simulink model "TransmissionController"  (Simulink 7.6)
settings: Solver=ode45  StartTime=0.0  StopTime=10.0  RelTol=1e-3
libraries: simulink x1
settings Model: Creator=Zsolt  LastModifiedBy=bapty
settings HardwareCC: TargetIntDivRoundTo=Zero  TargetEndianess=LittleEndian  TargetHWDeviceType=MATLAB Host  ProdEqTarget=off
settings RTWCC: SystemTargetFile=rsim.tlc  TemplateMakefile=rsim_default_tmf  Description=Rapid Simulation Target  ProcessScript=rsim_make_rtw_hook
settings RSimTargetCC: TargetFunctionLibrary=ANSI_C  ERTMultiwordTypeDef=System defined  ERTCodeCoverageTool=None  ERTMultiwordLength=256  IsPILTarget=off  EnableShiftOperators=on  PortableWordSizes=off

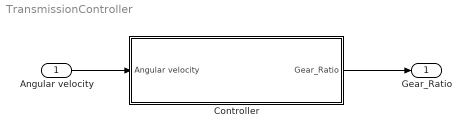
== system TransmissionController ==
  Angular velocity : Inport
  Controller : Subsystem
  Gear_Ratio : Outport
  wires:
  Angular velocity/1 -> Controller/1(Angular velocity)
  Controller/1(Gear_Ratio) -> Gear_Ratio/1

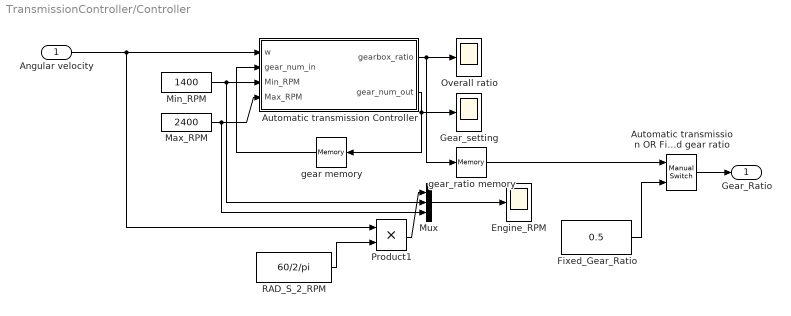
== system TransmissionController/Controller ==
  Angular velocity : Inport
  Automatic transmission Controller : Stateflow chart  TreatAsAtomicUnit=on
  Automatic transmission OR Fixed gear ratio : simulink/Signal Routing/Manual Switch  SystemSampleTime=-1  sw=0  action=0  varsize=off
  Engine_RPM : Scope
      settings: TimeRange=500  YMin=0  YMax=2500  SaveName=ScopeData18
  Fixed_Gear_Ratio : Constant  Value=0.5
  Gear_setting : Scope
      settings: TimeRange=500  YMin=0  SaveName=ScopeData17
  Max_RPM : Constant  Value=2400
  Min_RPM : Constant  Value=1400
  Mux : Mux  Inputs=3
  Overall ratio : Scope
      settings: TimeRange=500  YMin=0.04  YMax=0.12  SaveName=ScopeData16
  Product1 : Product  RndMeth=Zero
  RAD_S_2_RPM : Constant  Value=60/2/pi
  gear memory : Memory  X0=1
  gear_ratio memory : Memory  X0=1
  Gear_Ratio : Outport
  wires:
  RAD_S_2_RPM/1 -> Product1/2
  Product1/1 -> Mux/1
  Mux/1 -> Engine_RPM/1
  Max_RPM/1 -> Automatic transmission Controller/4(Max_RPM), Mux/3
  Min_RPM/1 -> Automatic transmission Controller/3(Min_RPM), Mux/2
  Automatic transmission Controller/1(gearbox_ratio) -> Overall ratio/1, gear_ratio memory/1
  gear memory/1 -> Automatic transmission Controller/2(gear_num_in)
  Automatic transmission Controller/2(gear_num_out) -> gear memory/1, Gear_setting/1
  Fixed_Gear_Ratio/1 -> Automatic transmission OR Fixed gear ratio/2
  gear_ratio memory/1 -> Automatic transmission OR Fixed gear ratio/1
  Automatic transmission OR Fixed gear ratio/1 -> Gear_Ratio/1
  Angular velocity/1 -> Automatic transmission Controller/1(w), Product1/1

== matlab function Controller/Automatic transmission Controller ==
  data: gearbox_ratio output double; w input double; gear_num_out output double; gear_num_in input double; Min_RPM input double; Max_RPM input double
function [gearbox_ratio, gear_num_out] = fcn(w, gear_num_in, Min_RPM, Max_RPM)
%#eml

%Min_RPM = 1400;
%Max_RPM = 2400;

gear_num_out = gear_num_in;
gearbox_ratio = 0.12/1;


if (w > (Max_RPM*2*pi/60)) && (gear_num_in < 4)
    gear_num_out = gear_num_in + 1;    
elseif (w < (Min_RPM*2*pi/60)) && (gear_num_in > 1)
    gear_num_out = gear_num_in - 1;
end

switch gear_num_out
    case 1
        gearbox_ratio = 0.12/3.5;
    case 2
        gearbox_ratio = 0.12/2.2;        
    case 3
        gearbox_ratio = 0.12/1.4;        
    case 4
        gearbox_ratio = 0.12/1;
end
